simulink model "AM_SIMPLE_5_2"  (R2024a)
settings: Solver=VariableStepAuto  StartTime=0.0  StopTime=30  RelTol=1e-3
settings Model: Creator=Braan  LastModifiedBy=Braan

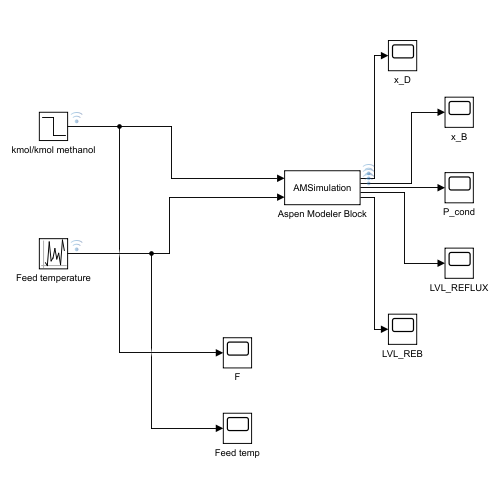
[thumbnail: Simulink's stored preview of the top-level diagram]
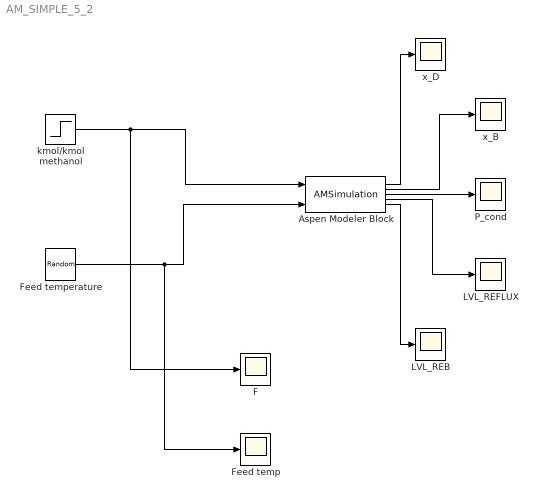
== system AM_SIMPLE_5_2 ==
  Aspen Modeler Block : M-S-Function  LoadFcn=|  FunctionName=AMSimulation  Parameters="'C:\\git\\master_project\\Aspen_files\\Distillation\\sim1_SIMPLE_5_2.dynf','AD Application',2,'STREAMS(\"F\").ZR(\"METHANOL\")|kmol/kmol\\STREAMS(\"F\").T|C',5,'STREAMS(\"D\").Zn(\"METHANOL\")|kmol/kmol\\STREAMS(\"B\").Zn(\"WATER\")|kmol/kmol\\BLOCKS(\"COLUMN\").Condenser(1).P|bar\\BLOCKS(\"COLUMN\").Stage(1).Level|m\\BLOCKS(\"COLUMN\").SumpLevel|m',true,true,true"
      | LoadModel=actxserver('AMSimulation.Control');                 
      | invoke(LoadModel,'LoadModel',get_param(gcb,'Parameters'),pwd);
      | LoadModel.delete;
      | rehash;
      settings: DeleteFcn=|
      | CloseModel=actxserver('AMSimulation.Control');
      | invoke(CloseModel,'CloseModel',get_param(gcb,'Parameters'));
      | CloseModel.delete;
      settings: OpenFcn=|
      | SetupGUI=actxserver('AMSimulation.Setup');
      | NewParam=invoke(SetupGUI,'SetupModel',get_param(gcb,'Parameters'),pwd,get_param(gcb,'Name'));
      | set_param(gcb,'Parameters',NewParam);
      | SetupGUI.delete;
  F : Scope
  Feed temp : Scope
  Feed temperature : UniformRandomNumber  Minimum=44  Maximum=48  Seed=1  SampleTime=0.1
  LVL_REB : Scope
  LVL_REFLUX : Scope
  P_cond : Scope
  kmol/kmol methanol : Step  Before=0.5  After=0.4  SampleTime=0
  x_B : Scope
  x_D : Scope
  wires:
  kmol/kmol methanol/1 -> F/1, Aspen Modeler Block/1
  Feed temperature/1 -> Feed temp/1, Aspen Modeler Block/2
  Aspen Modeler Block/3 -> P_cond/1
  Aspen Modeler Block/2 -> x_B/1
  Aspen Modeler Block/1 -> x_D/1
  Aspen Modeler Block/4 -> LVL_REFLUX/1
  Aspen Modeler Block/5 -> LVL_REB/1
